simulink model "CABLE_UNIT_TEST"  (Simulink 7.8)
settings: Solver=ode45  StartTime=0.0  StopTime=0.05  RelTol=1e-3
PostLoadFcn:
  | Ts=80e-6;
InitFcn:
  | Ts=80e-6;
libraries: powerlib x6, cables_lib x2, artemis x1
settings Model: ARTEMISmethode_block_infos=$$__separator__$$CABLE_UNIT_TEST/ARTEMIS Guide$$__separator__$$  Creator=re25624  LastModifiedBy=re25624

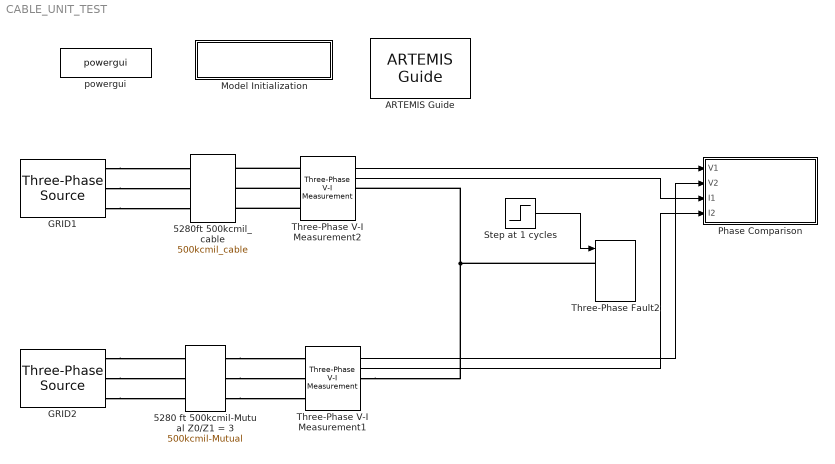
== system CABLE_UNIT_TEST ==
  5280 ft 500kcmil-Mutual Z0/Z1 = 3 : cables_lib/500kcmil-Mutual  length=5280  par_sets=1  ratio=3
  5280ft 500kcmil_cable : cables_lib/500kcmil_cable  length=5280  par_sets=1
  ARTEMIS Guide : artemis/ARTEMIS/ARTEMIS Guide  Tag=FTSSmethode_opal_4hx0r99  Description=5.0_z1  lock=on  Ts=Ts  opt=art5  dyna=off  nb_perm=4  RT_fullcomp=off  ssn=on  ssn_itvc=off  ssn_ivic=off  ssn_ext=off  ssn_solver=Art5 with Backward Euler nodal interface  ssn_impulse=off  ssn_quasimpulse=off  ssn_impulse_loop=2  paraExtinctionThy=off  Thy_Impulse=on  dtc=Off  dtc_opt=normal  ao=on  simtype=off  ct_mac=off  lin_mov=off  lsp=[0.001 2]  spike_skip=Disabled  dtc_extra=1  dtc_sws=normal  dtc_pied=0.5  SPSRulesBlock=SPSRules  tre=on  ctmm=off  LF=off  dpl_type=ARTEMiS DPL  rlc_type=off  custom_type=off  para=on  ssn_ImpulseLoopBlockedStateUpdate=2  ssn_mov_iter_number=5  ssn_switch_iter_number=5
  GRID1 : powerlib/Electrical Sources/Three-Phase Source  Voltage=13800  PhaseAngle=0  Frequency=60  InternalConnection=Yg  SpecifyImpedance=on  Resistance=0.8929  Inductance=16.58e-3  ShortCircuitLevel=375e6  BaseVoltage=13800  XRratio=7.9  BusType=swing  Pref=0  Qref=0  Qmin=-inf  Qmax=inf
  GRID2 : powerlib/Electrical Sources/Three-Phase Source  Voltage=13800  PhaseAngle=0  Frequency=60  InternalConnection=Yg  SpecifyImpedance=on  Resistance=0.8929  Inductance=16.58e-3  ShortCircuitLevel=375e6  BaseVoltage=13800  XRratio=7.9  BusType=swing  Pref=0  Qref=0  Qmin=-inf  Qmax=inf
  Model Initialization : Subsystem  AncestorBlock=artemis/Tools /Misc/Model Initialization  mask(Model Functions){InitFcnX=Ts=80e-6;, prel=off, posl=on, inif=on, strf=off}
      mask prompts: InitFcnX "Initialisation"; prel "Preload Function"; posl "PostLoad Function"; inif "InitFcn"; strf "StartFcn"
      mask init:
      | currentBlock = gcb;
      | root = bdroot(currentBlock);
      | 
      | if ~strcmp(get_param(root,'BlockDiagramType'),'library')
      |     if prel==1
      |         set_param(root, 'PreLoadFcn', InitFcnX);
      |     else
      |         set_param(root, 'PreLoadFcn', '');
      |     end
      |     if inif==1
      |         set_param(root, 'InitFcn', InitFcnX);
      |     else
      |         set_param(root, 'InitFcn', '');
      |     end
      |     if strf==1
      |         set_param(root, 'StartFcn', InitFcnX);
      |     else
      |         set_param(root, 'StartFcn', '');
      |     end
      |     if posl==1
      |         set_param(root, 'PostLoadFcn', InitFcnX);
      |     else
      |         set_param(root, 'PostLoadFcn', '');
      |     end
      | end
      | 
      | pos = get_param(currentBlock, 'Position');
      | width = pos(3) - pos(1); height = pos(4) - pos(2);
      | txt = [ upper(root) '\n' '- InitFcn. . . . . '  get_param(root, 'InitFcn') ];
      settings: CopyFcn=set_param(gcb,'LinkStatus','inactive')
      mask Display: text(5, height*0.5, txt, 'horizontalAlignment', 'left', 'verticalAlignment', 'middle') ;
  Phase Comparison : Subsystem
  Step at 1 cycles : Step  Time=1/60  SampleTime=Ts
  Three-Phase V-I Measurement1 : powerlib/Measurements/Three-Phase V-I Measurement  VoltageMeasurement=phase-to-ground  SetLabelV=off  LabelV=Vabc  Vpu=off  VpuLL=off  CurrentMeasurement=yes  SetLabelI=off  LabelI=Iabc  Ipu=off  Pbase=100e6  Vbase=500e3  OutputType=Complex  PhasorSimulation=off  PSBequivalent=0
  Three-Phase V-I Measurement2 : powerlib/Measurements/Three-Phase V-I Measurement  VoltageMeasurement=phase-to-ground  SetLabelV=off  LabelV=Vabc  Vpu=off  VpuLL=off  CurrentMeasurement=yes  SetLabelI=off  LabelI=Iabc  Ipu=off  Pbase=100e6  Vbase=500e3  OutputType=Complex  PhasorSimulation=off  PSBequivalent=0
  Three-Phase Fault2 : powerlib/Elements/Three-Phase Fault  FaultA=on  FaultB=off  FaultC=off  FaultResistance=1e-4  GroundFault=on  GroundResistance=1e-4  External=on  SwitchStatus=[1 0]  SwitchTimes=[ 1/60 3/60]  InitialStates=[0 0 0]  SnubberResistance=1e6  SnubberCapacitance=inf  Measurements=None
  powergui : powerlib/powergui  Priority=2  SimulationMode=Discrete  SolverType=Tustin  SampleTime=Ts  frequency=60  SPID=off  DisableSnubberDevices=off  DisableRonSwitches=off  DisableVfSwitches=off  SwTol=0  Interpol=off  DisplayEquations=off  FunctionMessages=off  frequencyindice=0  Pbase=100e6  ErrMax=1e-4  Iterations=50  UnitsV=kV  UnitsW=MW  echomessages=off  HookPort=off  EnableUseOfTLC=off  x0status=blocks  RestoreLinks=warning  ResistiveCurrentMeasurement=off  Frange=logspace(0,3,50)  Ylog=off  Xlog=off  ShowGrid=off  save=off  variable=ZData  structure=0  ZoomFFT=on  StartTime=0.0  cycles=2  DisplayStyle=off  fundamental=60  FreqAxis=off  MaxFrequency=1000  frequencyindicesteady=1  RmsSteady=1  display=off  Ts=0  methode=off
  wires:
  Three-Phase V-I Measurement2/1 -> Phase Comparison/1(V1)
  Three-Phase V-I Measurement1/1 -> Phase Comparison/2(V2)
  Three-Phase V-I Measurement1/2 -> Phase Comparison/4(I2)
  Step at 1 cycles/1 -> Three-Phase Fault2/1
  Three-Phase V-I Measurement2/2 -> Phase Comparison/3(I1)
  connections:
  GRID1/RConn3 -- 5280ft 500kcmil_cable/LConn3
  GRID1/RConn2 -- 5280ft 500kcmil_cable/LConn2
  GRID1/RConn1 -- 5280ft 500kcmil_cable/LConn1
  5280 ft 500kcmil-Mutual Z0/Z1 = 3/RConn3 -- Three-Phase V-I Measurement1/LConn3
  5280 ft 500kcmil-Mutual Z0/Z1 = 3/RConn2 -- Three-Phase V-I Measurement1/LConn2
  5280 ft 500kcmil-Mutual Z0/Z1 = 3/RConn1 -- Three-Phase V-I Measurement1/LConn1
  Three-Phase V-I Measurement2/LConn3 -- 5280ft 500kcmil_cable/RConn3
  Three-Phase V-I Measurement2/LConn2 -- 5280ft 500kcmil_cable/RConn2
  Three-Phase V-I Measurement2/LConn1 -- 5280ft 500kcmil_cable/RConn1
  Three-Phase Fault2/LConn1 -- Three-Phase V-I Measurement2/RConn1 -- Three-Phase V-I Measurement1/RConn1
  GRID2/RConn3 -- 5280 ft 500kcmil-Mutual Z0/Z1 = 3/LConn3
  GRID2/RConn2 -- 5280 ft 500kcmil-Mutual Z0/Z1 = 3/LConn2
  GRID2/RConn1 -- 5280 ft 500kcmil-Mutual Z0/Z1 = 3/LConn1

== system CABLE_UNIT_TEST/Model Initialization ==

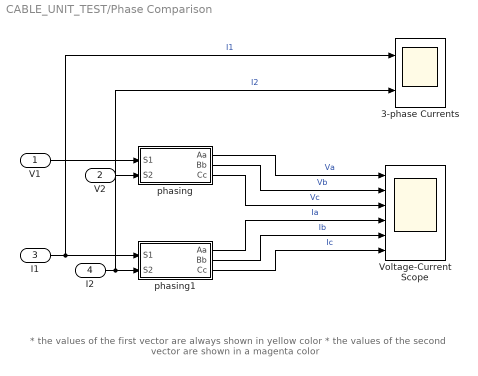
== system CABLE_UNIT_TEST/Phase Comparison ==
  note: * the values of the first vector are always shown in yellow color
      | * the values of the second vector are shown in a magenta color
  V1 : Inport
  V2 : Inport  Port=2
  I1 : Inport  Port=3
  I2 : Inport  Port=4
  3-phase Currents : Scope  NumInputPorts=2
      settings: TimeRange=0.05  YMin=-20000~-15000  YMax=25000~20000  SaveName=ScopeData2
  Voltage-Current Scope : Scope  NumInputPorts=6
      settings: TimeRange=0.05  YMin=-15000~-15000~-15000~-20000~-3e-012~-1  YMax=15000~15000~15000~30000~2e-012~1
  phasing : Subsystem
  phasing1 : Subsystem
  wires:
  phasing/1(Aa) -> Voltage-Current Scope/1  "Va"
  phasing/2(Bb) -> Voltage-Current Scope/2  "Vb"
  phasing/3(Cc) -> Voltage-Current Scope/3  "Vc"
  phasing1/1(Aa) -> Voltage-Current Scope/4  "Ia"
  phasing1/2(Bb) -> Voltage-Current Scope/5  "Ib"
  phasing1/3(Cc) -> Voltage-Current Scope/6  "Ic"
  V1/1 -> phasing/1(S1)
  V2/1 -> phasing/2(S2)
  I1/1 -> phasing1/1(S1), 3-phase Currents/1  "I1"
  I2/1 -> phasing1/2(S2), 3-phase Currents/2  "I2"

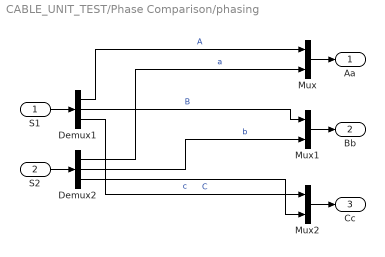
== system CABLE_UNIT_TEST/Phase Comparison/phasing ==
  S1 : Inport
  S2 : Inport  Port=2
  Demux1 : Demux  Outputs=3
  Demux2 : Demux  Outputs=3
  Mux : Mux  Inputs=2
  Mux1 : Mux  Inputs=2
  Mux2 : Mux  Inputs=2
  Aa : Outport
  Bb : Outport  Port=2
  Cc : Outport  Port=3
  wires:
  Demux1/1 -> Mux/1  "A"
  Demux2/1 -> Mux/2  "a"
  Demux1/2 -> Mux1/1  "B"
  Demux2/2 -> Mux1/2  "b"
  Demux1/3 -> Mux2/1  "C"
  Demux2/3 -> Mux2/2  "c"
  Mux/1 -> Aa/1
  S1/1 -> Demux1/1
  Mux1/1 -> Bb/1
  S2/1 -> Demux2/1
  Mux2/1 -> Cc/1

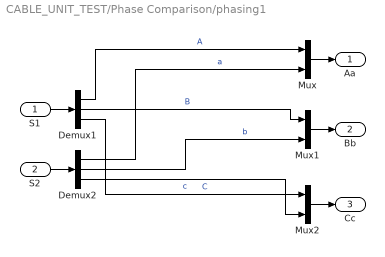
== system CABLE_UNIT_TEST/Phase Comparison/phasing1 ==
  S1 : Inport
  S2 : Inport  Port=2
  Demux1 : Demux  Outputs=3
  Demux2 : Demux  Outputs=3
  Mux : Mux  Inputs=2
  Mux1 : Mux  Inputs=2
  Mux2 : Mux  Inputs=2
  Aa : Outport
  Bb : Outport  Port=2
  Cc : Outport  Port=3
  wires:
  Demux1/1 -> Mux/1  "A"
  Demux2/1 -> Mux/2  "a"
  Demux1/2 -> Mux1/1  "B"
  Demux2/2 -> Mux1/2  "b"
  Demux1/3 -> Mux2/1  "C"
  Demux2/3 -> Mux2/2  "c"
  Mux/1 -> Aa/1
  S1/1 -> Demux1/1
  Mux1/1 -> Bb/1
  S2/1 -> Demux2/1
  Mux2/1 -> Cc/1
